simulink model "Full_AM_Demod_Modul"  (R2023a)
settings: Solver=VariableStepAuto  StartTime=0.0  StopTime=1  RelTol=1e-3
libraries: dspfdesign x1
settings Model: Creator=Pedro  LastModifiedBy=Pedro

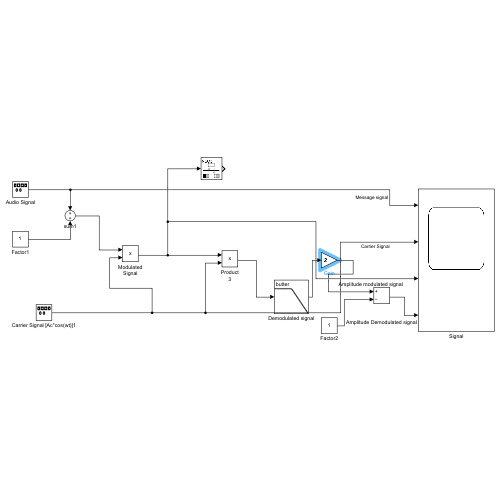
[thumbnail: Simulink's stored preview of the top-level diagram]
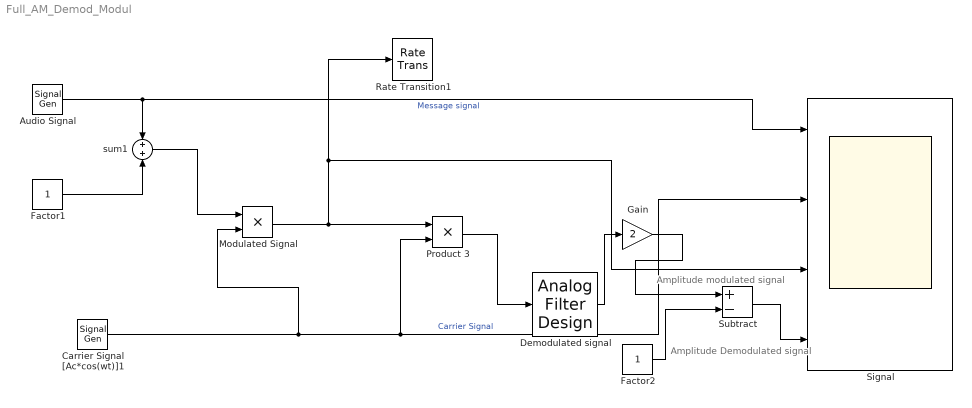
== system Full_AM_Demod_Modul ==
  note: Amplitude modulated signal
  note: Amplitude Demodulated signal
  Audio Signal : SignalGenerator  Frequency=20
  Carrier Signal [Ac*cos(wt)]1 : SignalGenerator  Frequency=110
  Demodulated signal : dspfdesign/Analog Filter Design  method=Butterworth  filttype=Lowpass  N=8  Wlo=2*pi*70  Whi=80  Rp=2  Rs=40
  Factor1 : Constant
  Factor2 : Constant
  Gain : Gain  Gain=2
  Modulated Signal : Product
  Product 3 : Product
  Rate Transition1 : RateTransition  OutPortSampleTime=0.0001
  Signal : Scope  NumInputPorts=4
  Subtract : Sum  Inputs=+-
  sum1 : Sum
  wires:
  Carrier Signal [Ac*cos(wt)]1/1 -> Signal/2, Product 3/2, Modulated Signal/2  "Carrier Signal"
  Modulated Signal/1 -> Product 3/1, Signal/3, Rate Transition1/1
  sum1/1 -> Modulated Signal/1
  Product 3/1 -> Demodulated signal/1
  Audio Signal/1 -> sum1/1, Signal/1  "Message signal"
  Factor1/1 -> sum1/2
  Demodulated signal/1 -> Gain/1
  Gain/1 -> Subtract/1
  Factor2/1 -> Subtract/2
  Subtract/1 -> Signal/4
